simulink model "final_19_2_24_hecho_por_mi_simulink"  (R2021a)
settings: Solver=VariableStepAuto  StartTime=0.0  StopTime=10.0  RelTol=1e-3
libraries: cstblocks x1
settings Model: Creator=pedro  LastModifiedBy=pedro

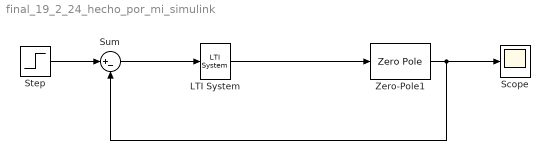
== system final_19_2_24_hecho_por_mi_simulink ==
  LTI System : cstblocks/LTI System  sys=Cd  IC=[]
  Scope : Scope
  Step : Step  After=2*180/pi  SampleTime=0
  Sum : Sum  Inputs=|+-
  Zero-Pole1 : ZeroPole  Zeros=[-2 -2]  Poles=[0 4 4]
  wires:
  Step/1 -> Sum/1
  Sum/1 -> LTI System/1
  LTI System/1 -> Zero-Pole1/1
  Zero-Pole1/1 -> Sum/2, Scope/1
